simulink model "CurrentLoop"  (R2014b)
settings: Solver=ode45  StartTime=0.0  StopTime=10  RelTol=1e-3
values from neighbouring files (symbols this model uses):
  H1 = Rs * (R4/R1) * 1/(R7+Rv2)    [InitModel.m]    (also in SystemModel.m = -(R4*Rs/R1) * 1/(R7+Rv2))
  R6 = 100e3    (= 100000)    [InitModel.m]    (also in SystemModel.m; SystemModel_marco.m)
  Vdc = 30    [InitModel.m]    (also in SystemModel.m; SystemModel_marco.m)
undefined symbols (not defined in the file or in its folder): sigbuilder_block
libraries: cstblocks x2
settings Model: Creator=Edoardo  LastModifiedBy=Edoardo

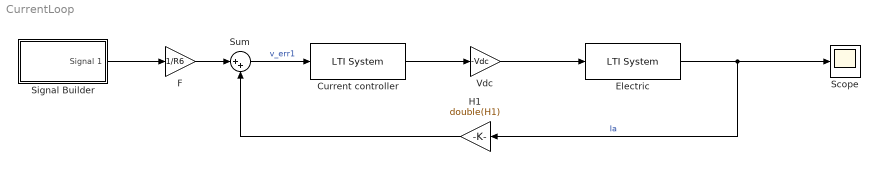
== system CurrentLoop ==
  Current controller : cstblocks/LTI System  sys=C1  IC=[]
  Electric : cstblocks/LTI System  sys=G1  IC=[]
  F : Gain  Gain=1/R6
  H1 : Gain  Gain=double(H1)
  Scope : Scope
      settings: YMin=-1  YMax=1
  Signal Builder : Subsystem  Tag=STV Subsys  LoadFcn=sigbuilder_block('load',[84 212.25 551.25 400.5 ]);  StartFcn=sigbuilder_block('start');  StopFcn=sigbuilder_block('stop');  ClipboardFcn=sigbuilder_block('clipboard');  mask(Sigbuilder block){}
      mask help: Simulink:masks:SigbuilderBlock_MD
      mask init:
      | if ~strcmp(get_param(bdroot(gcbh),'SimulationStatus'),'stopped') tuvar = sigbuilder_block('maskInit'); end
      settings: CopyFcn=sigbuilder_block('copy');  DeleteFcn=sigbuilder_block('delete');  ModelCloseFcn=sigbuilder_block('modelClose');  PreSaveFcn=sigbuilder_block('preSave');  PauseFcn=sigbuilder_block('pause');  ContinueFcn=sigbuilder_block('continue');  NameChangeFcn=sigbuilder_block('namechange');  OpenFcn=sigbuilder_block('open',[437.6 199.2 550.4 400 ]);  CloseFcn=sigbuilder_block('close');
      mask Display: plot(0, 0, 100, 100,[2, 2, 32, 32, 2], [68, 8, 8, 68, 68],[32, 2], [38, 38], [32, 19, 2],[53, 60, 44], [32, 17, 17, 2],[16, 16, 31, 31]);txt = getActiveGroup(gcbh);text(2, 100, txt,'verticalAlignment', 'top');
  Sum : Sum  Inputs=|++
  Vdc : Gain  Gain=-Vdc
  wires:
  Vdc/1 -> Electric/1
  Current controller/1 -> Vdc/1
  Electric/1 -> Scope/1, H1/1  "Ia"
  Sum/1 -> Current controller/1  "v_err1"
  H1/1 -> Sum/2
  F/1 -> Sum/1
  Signal Builder/1(Signal 1) -> F/1

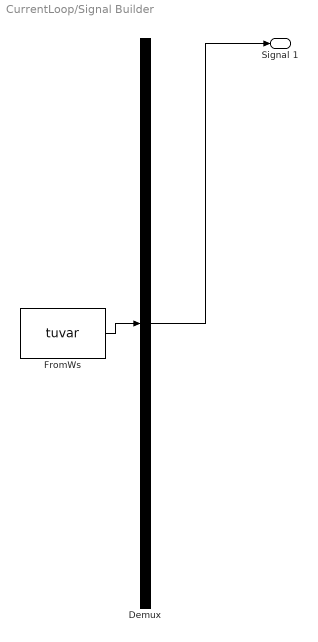
== system CurrentLoop/Signal Builder ==
  Demux : Demux  Tag=STV Demux  Outputs=1
  FromWs : FromWorkspace  Tag=STV FromWs  VariableName=tuvar  SampleTime=0
      SigBuilderData=|
      | common.afterFinalStr = 'Extrapolate'
      | common.sampleTime = 0
      | dataSet.timeRange = [0 10]
      | dataSet.name = 'Group 1'
      | sbobj.Groups.Name = 'Group 1'
      | sbobj.Groups.Signals.Name = 'Signal 1'
      | sbobj.Groups.Signals.XData = [0 0.05 10]
      | sbobj.Groups.Signals.YData = [0 1 1]
  Signal 1 : Outport  Tag=STV Outport
  wires:
  Demux/1 -> Signal 1/1
  FromWs/1 -> Demux/1
